simulink model "inverted_pendulum"  (R2024b)
settings: Solver=FixedStepAuto  StartTime=0.0  StopTime=10.0  FixedStep=0.0001  RelTol=1e-3
settings Model: Creator=JS  LastModifiedBy=JS

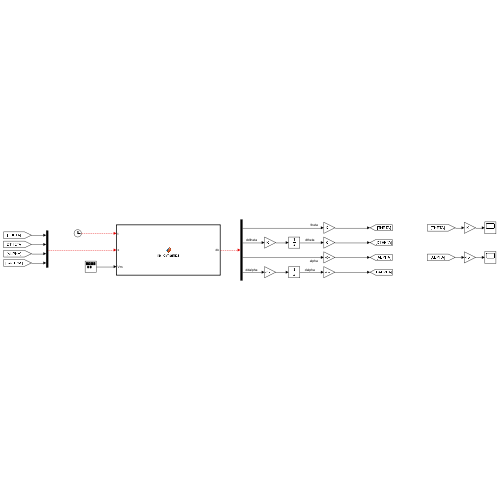
[thumbnail: Simulink's stored preview of the top-level diagram]
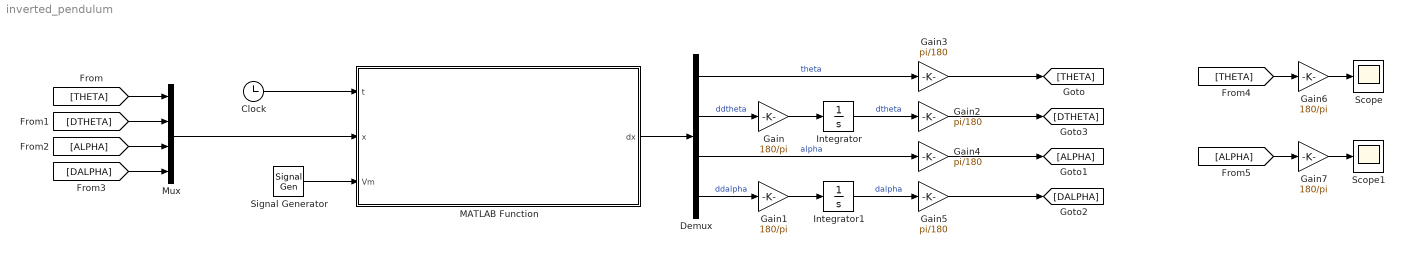
== system inverted_pendulum ==
  Clock : Clock
  Demux : Demux
  Gain{,1,6..7} (4 alike) : Gain  Gain=180/pi
  Gain{2..5} (4 alike) : Gain  Gain=pi/180
  Integrator : Integrator
  Integrator1 : Integrator
  MATLAB Function : MATLAB Function  TreatAsAtomicUnit=on
  Mux : Mux
  Scope : Scope
  Scope1 : Scope
  Signal Generator : SignalGenerator  WaveForm=sawtooth  Amplitude=20  Frequency=2*pi  Units=rad/sec
  wires:
  MATLAB Function/1(dx) -> Demux/1
  Demux/2 -> Gain/1  "ddtheta"
  Demux/4 -> Gain1/1  "ddalpha"
  Integrator/1 -> Gain2/1  "dtheta"
  Integrator1/1 -> Gain5/1  "dalpha"
  Demux/1 -> Gain3/1  "theta"
  Clock/1 -> MATLAB Function/1(t)
  Signal Generator/1 -> MATLAB Function/3(Vm)
  [DALPHA] -> Mux/4
  [DTHETA] -> Mux/2
  [THETA] -> Mux/1
  Mux/1 -> MATLAB Function/2(x)
  [ALPHA] -> Mux/3
  Gain1/1 -> Integrator1/1
  Gain/1 -> Integrator/1
  Gain2/1 -> [DTHETA]
  Gain3/1 -> [THETA]
  Gain5/1 -> [DALPHA]
  Gain4/1 -> [ALPHA]
  Demux/3 -> Gain4/1  "alpha"
  [THETA] -> Gain6/1
  Gain6/1 -> Scope/1
  Gain7/1 -> Scope1/1
  [ALPHA] -> Gain7/1

== matlab function inverted_pendulum/MATLAB Function ==
  data: t input; x input; Vm input; dx output
function dx = rip_dynamics(t, x, Vm)

% === Parameters ===
mp = 0.127; Lp = 0.337; lp = 0.156;
Jp = 0.0012 + mp*lp^2; Bp = 0.0024;

mr = 0.257; Lr = 0.216;
Jr = 0.0020; Br = 0.0024;

Kg = 70; km = 0.007; kt = 0.007; Rm = 2.6;
eta_m = 0.69; eta_g = 0.90; g = 9.81;

% === States ===
theta  = x(1);
dtheta = x(2);
alpha  = x(3);
dalpha = x(4);

% === Angle Limits ===
theta_limit = deg2rad(40);
theta = max(min(theta, theta_limit), -theta_limit);        % Clamp θ
alpha = mod(alpha + pi, 2*pi) - pi;                         % Wrap α

% === Motor Torque ===
tau = (eta_g * Kg * eta_m * kt * (Vm - Kg * km * dtheta)) / Rm;

% === Dynamics ===
c = cos(alpha); s = sin(alpha);

M11 = Jr + mp*Lr^2 + mp*lp^2 - mp*lp^2*c^2;
M12 = -mp * Lr * lp * c;
M21 = M12;
M22 = Jp + mp * lp^2;
M = [M11, M12; M21, M22];

RHS1 = tau - Br*dtheta + (mp*lp^2*s*c + mp*Lr*lp*s)*dalpha*dtheta;
RHS2 = -Bp*dalpha - mp*lp^2*c*s*dtheta^2 - mp*lp*g*s;
RHS = [RHS1; RHS2];

acc = M \ RHS;  % [thetaddot; alphaddot]

% === Output dx ===
dx = zeros(4,1);
dx(1) = dtheta;     % theta dot
dx(2) = acc(1);     % theta double dot
dx(3) = dalpha;     % alpha dot
dx(4) = acc(2);     % alpha double dot

end
